simulink model "Li_Slotine"  (R2021b)
(part 4 of 5)

et50 = qrd4.*(qd6.*(t1420-t1615+t1681+t1695+t1706+t1711+t1743+t1843)+qd3.*t2034+qd2.*t2082+qd1.*(t1185+t1194-t1259+t1260)+qd5.*(t1101+t1103+t1154+t1155+t1550+t1609+t1683+t1726+t1749+t1756+t1767+t1774+t1874+t1923+t1924+t1925)+qd4.*(t1793-t1876+t2034))+qrd6.*(t2058-t2110+qd2.*(t1589+t1643+t1649+t1706+t1711-t1736+t1743-t1778+t1881+t1912+t1917+t2016+t2018+(t8.*t914.*(t263+t456-t922-t978))./2.0)-qd5.*(et45+et46)+qd4.*(t1420+t1589-t1615+t1643+t1649+t1681+t1695+t1706+t1711+t1743+t1843+t1881+t1912+t1917+t2016+t2018)+qd3.*(t1589+t1643+t1649+t1881+t1912+t1917+t2016+t2018))+qrdd6.*(t1483+t1488+t1585+t1642+t1651+t1652)-qrdd5.*(t1514+t1517+t1586+t1636+t1637+t1730);
et51 = t230+t258+t267+qrd5.*(t2051+qd3.*(t552+t554+t664+t667+t1129+t1132+t1167+t1169+t1232+t1239+t1340+t1341+t1499+t1504+t1543+t1544+t1549+t1610+t1690+t1727+t1873+t1929+t1949+t1951)+qd2.*(t552+t554+t720+t723+t1129+t1132+t1167+t1169+t1232+t1239+t1340+t1341+t1499+t1504+t1549+t1561+t1564+t1639+t1727+t1761+t1893+t1929+t1949+t1951)+qd4.*(t551+t553+t1129+t1132+t1167+t1169+t1232+t1239+t1340+t1341+t1718+t1949+t1951)-qd5.*(t1096+t1102+t1270+t1347+t1353+t1442+t2094-t778.*t1593-t8.*t363.*t592+t2.*t363.*(t243-t422)))+qrd2.*(t1868-qd4.*t1978+qd3.*t2066+qd5.*(t552+t554+t720+t723+t1340+t1341+t1499+t1504+t1549+t1561+t1564+t1639+t1727+t1761+t1893+t1929)+qd2.*(t1134+t1138+t1699+t1367.*t1593+t1486.*t1509+t15.*t363.*t575+t17.*t363.*t575));
et52 = -qrd1.*(t1858+qd5.*(t689+t691-t787+t791+t1019-t1079+t1130+t1131-t1176-t1177+t1268-t1537-t1538+t1654+(t568.*(t426-t712))./2.0+(t1049.*(t424-t435-t609+t714))./2.0)+qd4.*(t533-t785-t1528+t1529)+qd3.*(t533-t785+t940-t941+t1041+t1050-t1528+t1529)+qd2.*(t533-t785-t985+t992+t1104+t1107-t1528+t1529))+qrdd3.*t1987+qrdd2.*t2009+qrdd4.*(t1199+t1201+t15.*t379+t17.*t379+t1593.^2)+qrdd1.*(t1109+t1222+t1223)-qrd4.*(qd3.*t1974+qd2.*t1978+qd4.*(t683+t684+t1133+t1139+t1796)-qd5.*(t551+t553+t1340+t1341+t1718));
et53 = qrd3.*(t1836+qd3.*(t781+t783+t1134+t1138+t1664+t1860+t1393.*t1452)-qd4.*t1974+qd2.*t2066+qd5.*(t552+t554+t664+t667+t1340+t1341+t1499+t1504+t1543+t1544+t1549+t1610+t1690+t1727+t1873+t1929))-qrdd5.*(t1118+t1164+t1171+t1226+t1229+t1833);
et54 = t1313+t1613+t1653-t1659+t1660+t1725+t1748+t1799+t1821+t1823+t1847+t1848+t1869-t1889+t2006-t2007+(t132.*(t590+t600-t958-t1017-t1018+t453.*(t61-t241).*8.084033333333334e-4))./2.0+(t172.*(t589+t602-t953-t1030-t1032+t452.*(t60-t192).*8.084033333333334e-4))./2.0;
et55 = (t12.*t29.*(t697+t945-t1211-t1213+t194.*(-t270-t294+t334+t337+t396+t2.*t25.*(t60-t192)).*8.084033333333334e-4+t238.*(-t269-t295+t352+t356+t385+t8.*t25.*(t61-t241)).*8.084033333333334e-4))./2.0+(t2.*t763.*(t444-t445-t639+t969))./2.0-(t6.*t29.*t1583)./2.0;
et56 = (t29.*t30.*(t779+t1253+t907.*(t61-t241).*8.084033333333334e-4))./2.0+(t2.*t491.*(t429-t960))./2.0+(t8.*t491.*(t446-t970))./2.0;
et57 = t1313+t1613+t1653-t1659+t1660+t1725+t1787+t1821+t1823+t1824+t1828+t1847+t1848+t1869-t1889+t2003+t2019+t2022+(t132.*(t590+t600-t958-t1017-t1018+t453.*(t61-t241).*8.084033333333334e-4))./2.0+(t172.*(t589+t602-t953-t1030-t1032+t452.*(t60-t192).*8.084033333333334e-4))./2.0+(t2.*t763.*(t444-t445-t639+t969))./2.0-(t6.*t29.*t1583)./2.0;
et58 = (t2.*t491.*(t429-t960))./2.0+(t8.*t491.*(t446-t970))./2.0;
et59 = t230+t257+t266-qrd5.*(t2085-qd3.*(t1101+t1103+t1154+t1155+t1548+t1588+t1609+t1640+t1647+t1689+t1726+t1747+t1752+t1770+t1776+t1872+t1879+t1904+t1908+t1923+t1924+t1928+t1994+t1995)-qd2.*(t1101+t1103+t1207+t1209+t1548+t1588+t1638+t1640+t1647+t1726+t1747+t1752+t1760+t1783+t1790+t1879+t1892+t1904+t1908+t1923+t1924+t1928+t1994+t1995)-qd4.*(t1086+t1087+t1588+t1640+t1647+t1717+t1879+t1904+t1908+t1923+t1924+t1994+t1995)+qd5.*(t1400+t1402-t1436+t1746+t1797+t1802+t1804+t1854+t1856-t1883+t1927+t1980+t1999+t2001-t777.*t1592+t2.*t29.*(t589+t602-t953-t1030-t1032+t452.*(t60-t192).*8.084033333333334e-4)-t8.*t763.*t877-t2.*t763.*t886)+qd6.*(et54+et55+et56));
et60 = qrd6.*(t2053-t2110+qd3.*(t1589+t1643+t1649+t1881+t1912+t1917+t2016+t2018+t2076)-qd5.*(et57+et58)+qd4.*(t1589+t1643+t1649+t1881+t1912+t1917+t2016+t2018)+qd2.*(t1429+t1589+t1643+t1649+t1669+t1679+t1693-t1736-t1778+t1842+t1881+t1912+t1917+t2016+t2018+(t8.*t914.*(t263+t456-t922-t978))./2.0));
et61 = qrd4.*(qd3.*t2042+qd2.*t2044+qd4.*(t1245+t1246+t1793+t1902+t1905)-qd5.*(-t1086-t1087+t1713+(t8.*(t589+t602-t953-t1030-t1032+t452.*(t60-t192).*8.084033333333334e-4))./2.0+(t2.*(t590+t600-t958-t1017-t1018+t453.*(t61-t241).*8.084033333333334e-4))./2.0));
et62 = -qrd1.*(t1891+t2070+qd5.*(t534+t547+t898+t904+t972+t974+t1007+t1012+t1137+t1299+t1300+t1316+t1401+t1406+t1418+t1430+t1739+t1742+t1810+t1815)+qd4.*t2026+qd3.*(t1185+t1194-t1259+t1260+t2026)+qd2.*(t1235+t1241-t1321+t1323+t2026))+qrdd2.*t2033+qrdd3.*t2032+qrd2.*(t1961-t2081+qd4.*t2044+qd3.*t2093+qd5.*(t1101+t1103+t1207+t1209+t1548+t1638+t1726+t1747+t1752+t1760+t1783+t1790+t1892+t1923+t1924+t1928)+qd2.*(-t1696+t1902+t1905+t1366.*t1592+t1485.*t1508+t15.*t763.*t921+t17.*t763.*t921))+qrdd1.*(t535+t1025+t1056+t1380+t1381)+qrdd4.*(t1621+t1622+t15.*t766+t17.*t766+t1592.^2)+qrd3.*(t1957+t2077+qd4.*t2042+qd2.*t2093+qd5.*(t1101+t1103+t1154+t1155+t1548+t1609+t1689+t1726+t1747+t1752+t1770+t1776+t1872+t1923+t1924+t1928)+qd3.*(t1303+t1305-t1662+t1859+t1902+t1905+t1392.*t1451))+qrdd6.*(t1454+t1461+t1585+t1651+t1652+t1763);
et63 = -qrdd5.*(t1473+t1475+t1586+t1636+t1637+t1832);
et64 = t1694+qd5.*(t12.*t25.*t68.*(-1.015540833333333e-3)+t6.*t29.*t615.*5.077704166666666e-4+t12.*t29.*t612.*5.077704166666666e-4+(t2.*t29.*t1046)./2.0+(t8.*t29.*(t604-t630))./2.0);
et65 = qd4.*(t689+t691+t706+t725-t813-t937+t956+t1077+t1078-t1116+t1130+t1131+t1268+t1654+(t568.*(t426-t712))./2.0+(t1049.*(t424-t435-t609+t714))./2.0)+qd3.*(t706+t725+t795+t802-t813-t937+t956+t1077+t1078-t1116+t1130+t1131+t1372+t1654+(t819.*(t426-t712))./2.0+(t1049.*(t424-t435-t609+t714))./2.0)+qd2.*(t706+t725-t813+t864+t871-t937+t956+t1077+t1078-t1116+t1130+t1131+t1408+t1654+(t888.*(t426-t712))./2.0+(t1049.*(t424-t435-t609+t714))./2.0);
et66 = -qrd2.*(t2061+t2101+qd3.*t2103+qd4.*t2112+qd2.*(t719+t722+t1340+t1341+t1631+t1946+t1947+t1187.*t1367+t1509.*t1567-t8.*t574.*(t424-t435-t609+t714)+t2.*t575.*t990-t2.*t574.*t1414-t8.*t575.*(t426-t712)))-t6.*t29.*5.675085e-1-qrd4.*(t2051+t2101+qd3.*t2108+qd2.*t2112+qd4.*(t551+t553+t1180+t1183+t1340+t1341+t1718+t1946+t1947+t994.*t1187+t1567.*t1593-t8.*t363.*(t424-t435-t609+t714)-t2.*t363.*t1414))+qrd1.*(et64+et65);
et67 = qrd5.*(qd2.*t2094+qd3.*t2094+qd4.*t2094+qd5.*(-t778.*t1187-(t25.*(t6.*t29.*t615.*1.015540833333333e-3+t12.*t29.*t612.*1.015540833333333e-3))./2.0+t990.*(t243-t422)+t592.*(t426-t712)+(t8.*t29.*t1445)./2.0+(t2.*t29.*(t981-t996))./2.0))-qrdd4.*(t1164+t1171+t1554+t1562+t1833)-qrdd3.*(t1237+t1242+t1554+t1562+t1731)-qrdd2.*(t1265+t1269+t1554+t1562+t1766)-qrdd1.*(t1463+t1466+t1491);
et68 = -qrd3.*(t2056+t2101+qd2.*t2103+qd4.*t2108+qd3.*(t663+t666+t1243+t1244+t1340+t1341+t1602+t1627+t1946+t1947+t1452.*t1567-t8.*t480.*(t424-t435-t609+t714)-t2.*t480.*t1414))+qrdd5.*((t426-t712).^2+t25.*t1491+t990.^2+t1187.^2+t2.*t29.*t1552+t8.*t29.*t1553);
et69 = t1313+t1613-t1659+t1725+t1748+t1799+t1821+t1823+t1847+t1848+t1869+t2006-t2007+(t8.*(t676+t913-t1285-t1467+t1278.*(t60-t192).*8.084033333333334e-4+t7.*t172.*(t291-t477+t172.*(t60-t192)).*8.084033333333334e-4))./2.0;
et70 = (t2.*(t687+t906-t1277-t1472+t1279.*(t61-t241).*8.084033333333334e-4+t7.*t132.*(t291-t477+t172.*(t60-t192)).*8.084033333333334e-4))./2.0;
et71 = (t12.*t29.*(t697+t945-t1211-t1213+t194.*(-t270-t294+t334+t337+t396+t2.*t25.*(t60-t192)).*8.084033333333334e-4+t238.*(-t269-t295+t352+t356+t385+t8.*t25.*(t61-t241)).*8.084033333333334e-4))./2.0+(t2.*t763.*(t444-t445-t639+t969))./2.0;
et72 = (t29.*t30.*(t779+t1253+t907.*(t61-t241).*8.084033333333334e-4))./2.0+(t2.*t491.*(t429-t960))./2.0+(t8.*t491.*(t446-t970))./2.0;
et73 = t1313+t1613-t1672+t1725+t1748+t1799+t1813+t1821+t1823+t1847+t1848+t2006-t2007+(t8.*(t676+t913-t1285-t1467+t1278.*(t60-t192).*8.084033333333334e-4+t7.*t172.*(t291-t477+t172.*(t60-t192)).*8.084033333333334e-4))./2.0;
et74 = (t2.*(t687+t906-t1277-t1472+t1279.*(t61-t241).*8.084033333333334e-4+t7.*t132.*(t291-t477+t172.*(t60-t192)).*8.084033333333334e-4))./2.0;
et75 = (t12.*t29.*(t697+t945-t1211-t1213+t194.*(-t270-t294+t334+t337+t396+t2.*t25.*(t60-t192)).*8.084033333333334e-4+t238.*(-t269-t295+t352+t356+t385+t8.*t25.*(t61-t241)).*8.084033333333334e-4))./2.0+(t2.*t863.*(t444-t445-t639+t969))./2.0;
et76 = (t29.*t30.*(t779+t1253+t907.*(t61-t241).*8.084033333333334e-4))./2.0+(t2.*t491.*(t429-t960))./2.0+(t8.*t491.*(t446-t970))./2.0;
et77 = t1313+t1613-t1688+t1725+t1748+t1799+t1821+t1823+t1837+t1847+t1848+t2006-t2007+(t8.*(t676+t913-t1285-t1467+t1278.*(t60-t192).*8.084033333333334e-4+t7.*t172.*(t291-t477+t172.*(t60-t192)).*8.084033333333334e-4))./2.0;
et78 = (t2.*(t687+t906-t1277-t1472+t1279.*(t61-t241).*8.084033333333334e-4+t7.*t132.*(t291-t477+t172.*(t60-t192)).*8.084033333333334e-4))./2.0;
et79 = (t12.*t29.*(t697+t945-t1211-t1213+t194.*(-t270-t294+t334+t337+t396+t2.*t25.*(t60-t192)).*8.084033333333334e-4+t238.*(-t269-t295+t352+t356+t385+t8.*t25.*(t61-t241)).*8.084033333333334e-4))./2.0+(t2.*t914.*(t444-t445-t639+t969))./2.0;
et80 = (t29.*t30.*(t779+t1253+t907.*(t61-t241).*8.084033333333334e-4))./2.0+(t2.*t491.*(t429-t960))./2.0+(t8.*t491.*(t446-t970))./2.0;
et81 = t6.*t1745-(t133.*t1780)./2.0-(t25.*t1975)./2.0+(t132.*t1963)./2.0+(t171.*(t779+t1253+t907.*(t61-t241).*8.084033333333334e-4))./2.0-(t172.*(t773-t790-t1089+t1203-t1214+t660.*(t60-t192).*8.084033333333334e-4))./2.0;
et82 = (t2.*t29.*(t676+t913-t1285-t1467+t1278.*(t60-t192).*8.084033333333334e-4+t7.*t172.*(t291-t477+t172.*(t60-t192)).*8.084033333333334e-4))./2.0;
et83 = t8.*t29.*(t687+t906-t1277-t1472+t1279.*(t61-t241).*8.084033333333334e-4+t7.*t132.*(t291-t477+t172.*(t60-t192)).*8.084033333333334e-4).*(-1.0./2.0)+(t12.*t29.*t1959)./2.0;
et84 = t1591-t1777+t1834+t1839-t1976+(t132.*(t687+t906-t1277-t1472+t1279.*(t61-t241).*8.084033333333334e-4+t7.*t132.*(t291-t477+t172.*(t60-t192)).*8.084033333333334e-4))./2.0;
et85 = (t172.*(t676+t913-t1285-t1467+t1278.*(t60-t192).*8.084033333333334e-4+t7.*t172.*(t291-t477+t172.*(t60-t192)).*8.084033333333334e-4))./2.0+t1522.*(t446-t970)-(t6.*t29.*t1775)./2.0;
et86 = t1313+t1613+t1653+t1660-t1688+t1725+t1748+t1799+t1821+t1823+t1837+t1847+t1848-t1889+t2006-t2007+(t132.*(t590+t600-t958-t1017-t1018+t453.*(t61-t241).*8.084033333333334e-4))./2.0+(t172.*(t589+t602-t953-t1030-t1032+t452.*(t60-t192).*8.084033333333334e-4))./2.0;
et87 = (t12.*t29.*(t697+t945-t1211-t1213+t194.*(-t270-t294+t334+t337+t396+t2.*t25.*(t60-t192)).*8.084033333333334e-4+t238.*(-t269-t295+t352+t356+t385+t8.*t25.*(t61-t241)).*8.084033333333334e-4))./2.0+(t2.*t914.*(t444-t445-t639+t969))./2.0-(t6.*t29.*t1583)./2.0;
et88 = (t29.*t30.*(t779+t1253+t907.*(t61-t241).*8.084033333333334e-4))./2.0+(t2.*t491.*(t429-t960))./2.0+(t8.*t491.*(t446-t970))./2.0;
et89 = t1313+t1613+t1653-t1659+t1660+t1725+t1748+t1799+t1821+t1823+t1847+t1848+t1869-t1889+t2006-t2007+(t132.*(t590+t600-t958-t1017-t1018+t453.*(t61-t241).*8.084033333333334e-4))./2.0+(t172.*(t589+t602-t953-t1030-t1032+t452.*(t60-t192).*8.084033333333334e-4))./2.0;
et90 = (t12.*t29.*(t697+t945-t1211-t1213+t194.*(-t270-t294+t334+t337+t396+t2.*t25.*(t60-t192)).*8.084033333333334e-4+t238.*(-t269-t295+t352+t356+t385+t8.*t25.*(t61-t241)).*8.084033333333334e-4))./2.0+(t2.*t763.*(t444-t445-t639+t969))./2.0-(t6.*t29.*t1583)./2.0;
et91 = (t29.*t30.*(t779+t1253+t907.*(t61-t241).*8.084033333333334e-4))./2.0+(t2.*t491.*(t429-t960))./2.0+(t8.*t491.*(t446-t970))./2.0;
et92 = t1313+t1613+t1653+t1660-t1672+t1725+t1748+t1799+t1813+t1821+t1823+t1847+t1848-t1889+t2006-t2007+(t132.*(t590+t600-t958-t1017-t1018+t453.*(t61-t241).*8.084033333333334e-4))./2.0+(t172.*(t589+t602-t953-t1030-t1032+t452.*(t60-t192).*8.084033333333334e-4))./2.0;
et93 = (t12.*t29.*(t697+t945-t1211-t1213+t194.*(-t270-t294+t334+t337+t396+t2.*t25.*(t60-t192)).*8.084033333333334e-4+t238.*(-t269-t295+t352+t356+t385+t8.*t25.*(t61-t241)).*8.084033333333334e-4))./2.0+(t2.*t863.*(t444-t445-t639+t969))./2.0-(t6.*t29.*t1583)./2.0;
et94 = (t29.*t30.*(t779+t1253+t907.*(t61-t241).*8.084033333333334e-4))./2.0+(t2.*t491.*(t429-t960))./2.0+(t8.*t491.*(t446-t970))./2.0;
et95 = t194.*t660.*(-4.042016666666667e-4)+t238.*t661.*4.042016666666667e-4-(t25.*t1168)./2.0+(t6.*t29.*t615)./1.0e+4+(t12.*t29.*t612)./1.0e+4-t12.*t39.*t896.*4.042016666666667e-4;
et96 = t12.*t40.*t907.*4.042016666666667e-4+(t8.*t29.*t1677)./2.0+(t2.*t29.*(t326-t350+t726-t727-t755+t12.*t39.*(t60-t192).*8.084033333333334e-4))./2.0;
et97 = -t1844-t2068+qd4.*(t709+t950+t1013+t1015-t1210-t1212+t1290+t1296-t1418+t1428+t1691+t1692-t1810-t1815+t194.*(-t270-t294+t334+t337+t396+t2.*t25.*(t60-t192)).*4.042016666666667e-4+t238.*(-t269-t295+t352+t356+t385+t8.*t25.*(t61-t241)).*4.042016666666667e-4);
et98 = qd3.*(t709+t950+t1088+t1097-t1210-t1212+t1290+t1296-t1487+t1493+t1691+t1692-t1810-t1815+t194.*(-t270-t294+t334+t337+t396+t2.*t25.*(t60-t192)).*4.042016666666667e-4+t238.*(-t269-t295+t352+t356+t385+t8.*t25.*(t61-t241)).*4.042016666666667e-4);
et99 = qd2.*(t709+t950+t1121+t1124-t1210-t1212+t1290+t1296-t1531+t1533+t1691+t1692-t1810-t1815+t194.*(-t270-t294+t334+t337+t396+t2.*t25.*(t60-t192)).*4.042016666666667e-4+t238.*(-t269-t295+t352+t356+t385+t8.*t25.*(t61-t241)).*4.042016666666667e-4)+qd5.*(et95+et96);
et100 = qrd6.*(t2046+qd4.*(et69+et70+et71+et72)+qd3.*(et73+et74+et75+et76)+qd2.*(et77+et78+et79+et80)+qd5.*(et81+et82+et83)+qd6.*(et84+et85))-t6.*t29.*1.356723+qrd5.*(qd2.*(t1746+t1797+t1802+t1804+t1854+t1856+t1980+t1999+t2001)+qd3.*(t1746+t1797+t1802+t1804+t1854+t1856+t1980+t1999+t2001)+qd4.*(t1746+t1797+t1802+t1804+t1854+t1856+t1980+t1999+t2001)-qd5.*(t777.*t1186-(t25.*t1959)./2.0+t877.*t1238+t886.*t1234+(t2.*t29.*(t773-t790-t1089+t1203-t1214+t660.*(t60-t192).*8.084033333333334e-4))./2.0+(t8.*t29.*t1963)./2.0));
et101 = qrdd6.*(-t1507+t172.*t1780-t132.*(t779+t1253+t907.*(t61-t241).*8.084033333333334e-4)+t1234.*(t429-t960)+t1238.*(t446-t970)+t12.*t29.*t1732)+qrd2.*(t2091+t2117-qd3.*t2113-qd4.*t2115-qd2.*(t1190+t1192+t1630+t1923+t1924+t1991+t1992+t1186.*t1366+t1508.*t1566+t2.*t921.*t1234+t8.*t921.*t1238-t2.*t914.*t1612-t8.*t914.*t1608)+qd6.*(et86+et87+et88))-qrdd3.*(t1514+t1517+t1730+t1791+t1795)-qrdd4.*(t1473+t1475+t1791+t1795+t1832)-qrdd2.*(t1539+t1541+t1765+t1791+t1795);
et102 = qrdd5.*(t25.*t1732+t1186.^2+t1234.^2+t1238.^2+t2.*t29.*t1780+t8.*t29.*(t779+t1253+t907.*(t61-t241).*8.084033333333334e-4))-qrdd1.*(t1577+t1578+t1732)+qrd4.*(t2085+t2117-qd2.*t2115-qd3.*t2114-qd4.*(t1086+t1087+t1481+t1482+t1717+t1923+t1924+t1991+t1992+t993.*t1186+t1566.*t1592-t2.*t763.*t1612-t8.*t763.*t1608)+qd6.*(et89+et90+et91))+qrd3.*(t2088+t2117-qd2.*t2113-qd4.*t2114-qd3.*(t1140+t1141+t1520+t1526+t1601+t1626+t1923+t1924+t1991+t1992+t1451.*t1566-t2.*t863.*t1612-t8.*t863.*t1608)+qd6.*(et92+et93+et94))-qrd1.*(et97+et98+et99);
et103 = t777.*t915+t25.*t1975+t1186.*t1371-t1238.*t1522-t886.*(t429-t960)-t877.*(t446-t970)+t1234.*(t444-t445-t639+t969)-t2.*t29.*(t676+t913-t1285-t1467+t1278.*(t60-t192).*8.084033333333334e-4+t7.*t172.*(t291-t477+t172.*(t60-t192)).*8.084033333333334e-4);
et104 = t8.*t29.*(t687+t906-t1277-t1472+t1279.*(t61-t241).*8.084033333333334e-4+t7.*t132.*(t291-t477+t172.*(t60-t192)).*8.084033333333334e-4);
et105 = t1591-t1777+t1834+t1839-t1976+(t132.*(t687+t906-t1277-t1472+t1279.*(t61-t241).*8.084033333333334e-4+t7.*t132.*(t291-t477+t172.*(t60-t192)).*8.084033333333334e-4))./2.0;
et106 = (t172.*(t676+t913-t1285-t1467+t1278.*(t60-t192).*8.084033333333334e-4+t7.*t172.*(t291-t477+t172.*(t60-t192)).*8.084033333333334e-4))./2.0+t1522.*(t446-t970)-(t6.*t29.*t1775)./2.0;
et107 = t1313+t1611-t1659+t1721+t1784+t1820+t1822+t1825+t1826+t1851+t1852+t1869+t2004+t2020+t2021+(t8.*(t676+t913-t1285-t1467+t1278.*(t60-t192).*8.084033333333334e-4+t7.*t172.*(t291-t477+t172.*(t60-t192)).*8.084033333333334e-4))./2.0;
et108 = (t2.*(t687+t906-t1277-t1472+t1279.*(t61-t241).*8.084033333333334e-4+t7.*t132.*(t291-t477+t172.*(t60-t192)).*8.084033333333334e-4))./2.0+(t2.*t763.*(t444-t445-t639+t969))./2.0+(t2.*t491.*(t429-t960))./2.0+(t8.*t491.*(t446-t970))./2.0;
et109 = t1313+t1611-t1672+t1721+t1784+t1813+t1820+t1822+t1825+t1826+t1851+t1852+t2004+t2020+t2021+(t8.*(t676+t913-t1285-t1467+t1278.*(t60-t192).*8.084033333333334e-4+t7.*t172.*(t291-t477+t172.*(t60-t192)).*8.084033333333334e-4))./2.0;
et110 = (t2.*(t687+t906-t1277-t1472+t1279.*(t61-t241).*8.084033333333334e-4+t7.*t132.*(t291-t477+t172.*(t60-t192)).*8.084033333333334e-4))./2.0+(t2.*t863.*(t444-t445-t639+t969))./2.0+(t2.*t491.*(t429-t960))./2.0+(t8.*t491.*(t446-t970))./2.0;
et111 = t1313+t1611-t1688+t1721+t1784+t1820+t1822+t1825+t1826+t1837+t1851+t1852+t2004+t2020+t2021+(t8.*(t676+t913-t1285-t1467+t1278.*(t60-t192).*8.084033333333334e-4+t7.*t172.*(t291-t477+t172.*(t60-t192)).*8.084033333333334e-4))./2.0;
et112 = (t2.*(t687+t906-t1277-t1472+t1279.*(t61-t241).*8.084033333333334e-4+t7.*t132.*(t291-t477+t172.*(t60-t192)).*8.084033333333334e-4))./2.0+(t2.*t914.*(t444-t445-t639+t969))./2.0+(t2.*t491.*(t429-t960))./2.0+(t8.*t491.*(t446-t970))./2.0;
et113 = t1313+t1611-t1672+t1721+t1784+t1813+t1820+t1822+t1825+t1826+t1851+t1852+t2004+t2020+t2021+(t8.*(t676+t913-t1285-t1467+t1278.*(t60-t192).*8.084033333333334e-4+t7.*t172.*(t291-t477+t172.*(t60-t192)).*8.084033333333334e-4))./2.0;
et114 = (t2.*(t687+t906-t1277-t1472+t1279.*(t61-t241).*8.084033333333334e-4+t7.*t132.*(t291-t477+t172.*(t60-t192)).*8.084033333333334e-4))./2.0+(t2.*t863.*(t444-t445-t639+t969))./2.0+(t2.*t491.*(t429-t960))./2.0+(t8.*t491.*(t446-t970))./2.0;
et115 = t1313+t1611-t1688+t1721+t1784+t1820+t1822+t1825+t1826+t1837+t1851+t1852+t2004+t2020+t2021+(t8.*(t676+t913-t1285-t1467+t1278.*(t60-t192).*8.084033333333334e-4+t7.*t172.*(t291-t477+t172.*(t60-t192)).*8.084033333333334e-4))./2.0;
et116 = (t2.*(t687+t906-t1277-t1472+t1279.*(t61-t241).*8.084033333333334e-4+t7.*t132.*(t291-t477+t172.*(t60-t192)).*8.084033333333334e-4))./2.0+(t2.*t914.*(t444-t445-t639+t969))./2.0+(t2.*t491.*(t429-t960))./2.0+(t8.*t491.*(t446-t970))./2.0;
et117 = t1591-t1777+t1834+t1839-t1976+(t132.*(t687+t906-t1277-t1472+t1279.*(t61-t241).*8.084033333333334e-4+t7.*t132.*(t291-t477+t172.*(t60-t192)).*8.084033333333334e-4))./2.0;
et118 = (t172.*(t676+t913-t1285-t1467+t1278.*(t60-t192).*8.084033333333334e-4+t7.*t172.*(t291-t477+t172.*(t60-t192)).*8.084033333333334e-4))./2.0+t1522.*(t446-t970)-(t6.*t29.*t1775)./2.0;
et119 = t1313+t1611-t1659+t1721+t1784+t1820+t1822+t1825+t1826+t1851+t1852+t1869+t2004+t2020+t2021+(t8.*(t676+t913-t1285-t1467+t1278.*(t60-t192).*8.084033333333334e-4+t7.*t172.*(t291-t477+t172.*(t60-t192)).*8.084033333333334e-4))./2.0;
et120 = (t2.*(t687+t906-t1277-t1472+t1279.*(t61-t241).*8.084033333333334e-4+t7.*t132.*(t291-t477+t172.*(t60-t192)).*8.084033333333334e-4))./2.0+(t2.*t763.*(t444-t445-t639+t969))./2.0+(t2.*t491.*(t429-t960))./2.0+(t8.*t491.*(t446-t970))./2.0;
et121 = qrdd6.*((t429-t960).^2+(t446-t970).^2+t172.*t1816+t915.^2-t132.*(-t675+t1009.*(t61-t241).*8.084033333333334e-4+t345.*(t291-t477+t172.*(t60-t192)).*8.084033333333334e-4)+t12.*t29.*t1775)-qrd5.*(t2046-qd5.*(et103+et104)+qd6.*(et105+et106)+qd4.*(et107+et108)+qd3.*(et109+et110)+qd2.*(et111+et112));
et122 = qrd3.*(t2059+t2110+qd2.*t2102+qd4.*t2106+qd3.*(t1484+t1494+t1569+t2012+t2015+t1451.*(t387+t473+t478+t26.*t29.*t132.*1.383e-1)-t8.*t863.*(t263+t456-t922-t978)+t2.*t863.*t1571)-qd5.*(et113+et114))+qrd2.*(-t2065+t2110+qd3.*t2102+qd4.*t2107+qd2.*(t2012+t2015+t915.*t1366+t1508.*(t387+t473+t478+t26.*t29.*t132.*1.383e-1)-t8.*t914.*(t263+t456-t922-t978)+t2.*t914.*t1571-t2.*t921.*(t429-t960)-t8.*t921.*(t446-t970))-qd5.*(et115+et116));
et123 = qrdd5.*(-t1507+t25.*t1775+t1234.*(t429-t960)+t1238.*(t446-t970)+t8.*t29.*(-t675+t1009.*(t61-t241).*8.084033333333334e-4+t345.*(t291-t477+t172.*(t60-t192)).*8.084033333333334e-4)+t2.*t29.*t1816)-qrdd1.*(t1775+t1051.*(t429-t960)+t1048.*(t446-t970));
et124 = -qrd1.*(qd4.*t2052+qd3.*t2057+qd2.*t2064-qd5.*(-t614+t869-t1249+t1443-t1449+t1733+t1734+(t380.*(t429-t960))./2.0+(t372.*(t446-t970))./2.0+t12.*t39.*(t291-t477+t172.*(t60-t192)).*4.042016666666667e-4));
et125 = -qrdd4.*(-t1763-t1818+t2.*(-t675+t1009.*(t61-t241).*8.084033333333334e-4+t345.*(t291-t477+t172.*(t60-t192)).*8.084033333333334e-4)+t2.*t763.*(t429-t960)+t8.*t763.*(t446-t970));
et126 = -qrdd3.*(-t1642-t1818+t2.*(-t675+t1009.*(t61-t241).*8.084033333333334e-4+t345.*(t291-t477+t172.*(t60-t192)).*8.084033333333334e-4)+t2.*t863.*(t429-t960)+t8.*t863.*(t446-t970));
et127 = -qrdd2.*(-t1674-t1818+t2.*(-t675+t1009.*(t61-t241).*8.084033333333334e-4+t345.*(t291-t477+t172.*(t60-t192)).*8.084033333333334e-4)+t2.*t914.*(t429-t960)+t8.*t914.*(t446-t970))+qrd6.*(qd2.*t2109+qd3.*t2109+qd4.*t2109-qd5.*(et117+et118));
et128 = qrd4.*(t2054+t2110+qd2.*t2107+qd3.*t2106+qd4.*(t1457+t1462+t2012+t2015+t915.*t993+t1592.*(t387+t473+t478+t26.*t29.*t132.*1.383e-1)-t8.*t763.*(t263+t456-t922-t978)+t2.*t763.*t1571)-qd5.*(et119+et120));
mt1 = [qrdd1.*(t15.*4.0513225e-3+t17.*4.0513225e-3+1.450440833333333e-3),0.0,0.0,0.0,0.0,0.0,-qrdd2.*t668-qrd2.*(qd2.*(t75.*t253+t71.*t261)-qd1.*(t377-t9.*t279.*(1.53e+2./2.5e+2)))+qrdd1.*(t18.*3.1312e-2+t3.^2.*3.1312e-2+t253.^2+t261.^2)+qd2.*qrd1.*(t377-t9.*t279.*(1.53e+2./2.5e+2))];
mt2 = [t127-qrdd1.*t668+qrdd2.*(t213+t214+t15.*t18.*3.74544e-1+t17.*t18.*3.74544e-1+t529.^2)-qd1.*qrd1.*(t377-t9.*t279.*(1.53e+2./2.5e+2))+qd2.*qrd2.*(-t529.*(t15.*t63+t17.*t63)+t3.*t9.*t15.*3.74544e-1+t3.*t9.*t17.*3.74544e-1),0.0,0.0,0.0,0.0];
mt3 = [-qrd3.*(t959+qd1.*t955+qd2.*t954)-qrdd3.*t948-qrdd2.*t1076-qrd2.*(t959+qd1.*t1067+qd2.*(t2.*t276.*t409+t8.*t276.*t403))-qrd1.*(qd3.*t955+qd2.*t1067)+qrdd1.*(t31.*2.739394083333334e-2+t20.^2.*2.739394083333334e-2+t403.^2+t409.^2)];
mt4 = [t127+t222-qrdd1.*t1076+qrdd3.*t1604+qrd2.*(qd3.*t1376+qd2.*(-t561.*t797+t15.*t276.*t277+t17.*t276.*t277))+qrdd2.*(t213+t214+t15.*t302+t17.*t302+t797.^2)+qrd3.*(qd2.*t1376+qd3.*(-t1128+t1376+t947.*(t2.*(t298-t2.*t9.*(1.53e+2./2.5e+2))+t8.*(t301-t8.*t9.*(1.53e+2./2.5e+2)))))+qd1.*qrd1.*t1067];
mt5 = [t222-qrdd1.*t948+qrdd2.*t1604+qrd3.*(qd2.*t1480+qd3.*(t331+t338-t1128))+qrdd3.*(t213+t214+t15.*t31.*3.2752729e-1+t17.*t31.*3.2752729e-1+t947.^2)+qrd2.*(qd3.*t1480+qd2.*(t1016-t797.*(t2.*(t298-t2.*t9.*(1.53e+2./2.5e+2))+t8.*(t301-t8.*t9.*(1.53e+2./2.5e+2)))+t179.*t276+t180.*t276-t561.*t947))+qd1.*qrd1.*t955,0.0,0.0,0.0];
mt6 = [-qrd3.*(-t1582+qd4.*t1600+qd2.*t1922+qd3.*(t933+t934-t8.*t347.*t500+t2.*t347.*t507))+qrdd4.*t1312+qrdd3.*t1391+qrdd2.*t1438+qrd2.*(t1617+qd2.*(-t2.*t408.*t596+t8.*t408.*t595+t2.*t423.*t696+t8.*t423.*t704)-qd4.*t1625-qd3.*t1922)+qrdd1.*(t35./5.0e+3+t36.*2.338600833333333e-3+t696.^2+t704.^2)-qrd4.*(-t1440+qd4.*(t845+t848)+qd3.*t1600+qd2.*t1625)+qrd1.*(qd4.*t1435+qd3.*t1579+qd2.*t1614)];
mt7 = [t127+t222+t231-qrd1.*(t1617-qd4.*t1184+qd3.*t1698)+qrdd1.*t1438+qrdd3.*t1884+qrdd4.*t1918+qrdd2.*(t513+t514+t15.*t432+t17.*t432+t1197.^2)-qrd3.*(t1704+t1762+qd2.*t1757-qd4.*(t1266+t1360+t1580+t1607-t15.*t29.*t408.*8.195e-2-t17.*t29.*t408.*8.195e-2))-qrd2.*(t1762+qd4.*t1595-qd2.*(t1059.*t1197+t15.*t408.*t423+t17.*t408.*t423))+qrd4.*(t1200-qd2.*t1595+qd3.*(t1266+t1360+t1580+t1607-t15.*t29.*t408.*8.195e-2-t17.*t29.*t408.*8.195e-2)-qd4.*(t1468+t1595+t1283.*(t908-t909)))];
mt8 = [t222+t231-qrd1.*(t1582+qd4.*t1083-qd2.*t1698)-qrd3.*(t1682+qd4.*t1540+qd2.*t1678)+qrdd1.*t1391+qrdd2.*t1884+qrdd4.*t1885+qrdd3.*(t513+t514+t15.*t358+t17.*t358+t1085.^2)+qrd2.*(-t1682+t1704+qd4.*(t1266+t1360+t1581+t1603+t15.*t144.*t347+t17.*t144.*t347)+qd2.*(t1059.*t1085+t15.*t347.*t423+t17.*t347.*t423))-qrd4.*(t1091+qd3.*t1540-qd2.*(t1266+t1360+t1581+t1603+t15.*t144.*t347+t17.*t144.*t347)+qd4.*(t1468+t1540+t1113.*(t908-t909)))];
mt9 = [t231-qrd2.*(t1200+qd4.*t1812+qd3.*t2029-qd2.*(t1355+t215.*t423+t216.*t423+t1197.*t1283+t1059.*(t908-t909)))-qrd1.*(t1440-qd3.*t1083+qd2.*t1184)+qrdd1.*t1312+qrdd3.*t1885+qrdd2.*t1918-qrd4.*(qd3.*t1755+qd2.*t1812+qd4.*(t346+t348+t1468))-qrd3.*(-t1091+qd4.*t1755+qd2.*t2029+qd3.*(t503+t504+t1257+t1597-t1085.*t1113))+qrdd4.*(t513+t514+(t908-t909).^2+t15.*t35.*6.7158025e-3+t17.*t35.*6.7158025e-3),0.0,0.0,et12+et13,et29+et30,et40+et41,et51+et52+et53,et66+et67+et68,0.0,et26+et27+et28,et36+et37+et38+et39,et47+et48+et49+et50,et59+et60+et61+et62+et63];
mt10 = [et100+et101+et102,et121+et122+et123+et124+et125+et126+et127+et128];
Yr = reshape([mt1,mt2,mt3,mt4,mt5,mt6,mt7,mt8,mt9,mt10],6,6);
end
